simulink model "ejercicio2"  (R2018a)
settings: Solver=VariableStepAuto  StartTime=0.0  StopTime=20.0  RelTol=1e-3
settings Model: Creator=OSCAR  LastModifiedBy=OSCAR

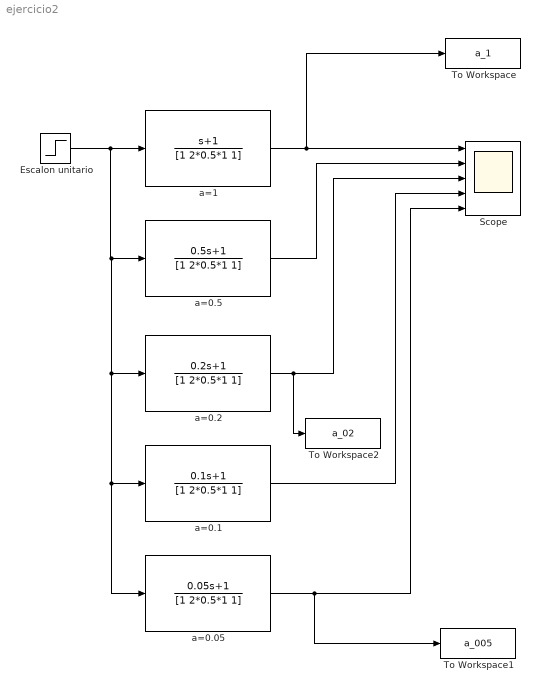
== system ejercicio2 ==
  Escalon unitario : Step  SampleTime=0.01
  Scope : Scope  NumInputPorts=5
  To Workspace : ToWorkspace  VariableName=a_1  SampleTime=-1
  To Workspace1 : ToWorkspace  VariableName=a_005  SampleTime=-1
  To Workspace2 : ToWorkspace  VariableName=a_02  SampleTime=-1
  a=0.05 : TransferFcn  Numerator=[0.05 1]  Denominator=[1 2*0.5*1 1]
  a=0.1 : TransferFcn  Numerator=[0.1 1]  Denominator=[1 2*0.5*1 1]
  a=0.2 : TransferFcn  Numerator=[0.2 1]  Denominator=[1 2*0.5*1 1]
  a=0.5 : TransferFcn  Numerator=[0.5 1]  Denominator=[1 2*0.5*1 1]
  a=1 : TransferFcn  Numerator=[1 1]  Denominator=[1 2*0.5*1 1]
  wires:
  Escalon unitario/1 -> a=0.05/1, a=0.1/1, a=0.2/1, a=0.5/1, a=1/1
  a=1/1 -> To Workspace/1, Scope/1
  a=0.5/1 -> Scope/2
  a=0.2/1 -> To Workspace2/1, Scope/3
  a=0.1/1 -> Scope/4
  a=0.05/1 -> To Workspace1/1, Scope/5
